simulink model "Simulation"  (R2015b)
settings: Solver=VariableStepAuto  StartTime=0.0  StopTime=10  RelTol=1e-3
undefined symbols (not defined in the file or in its folder): sigbuilder_block
settings Model: Creator=TOSHIBA  LastModifiedBy=TOSHIBA

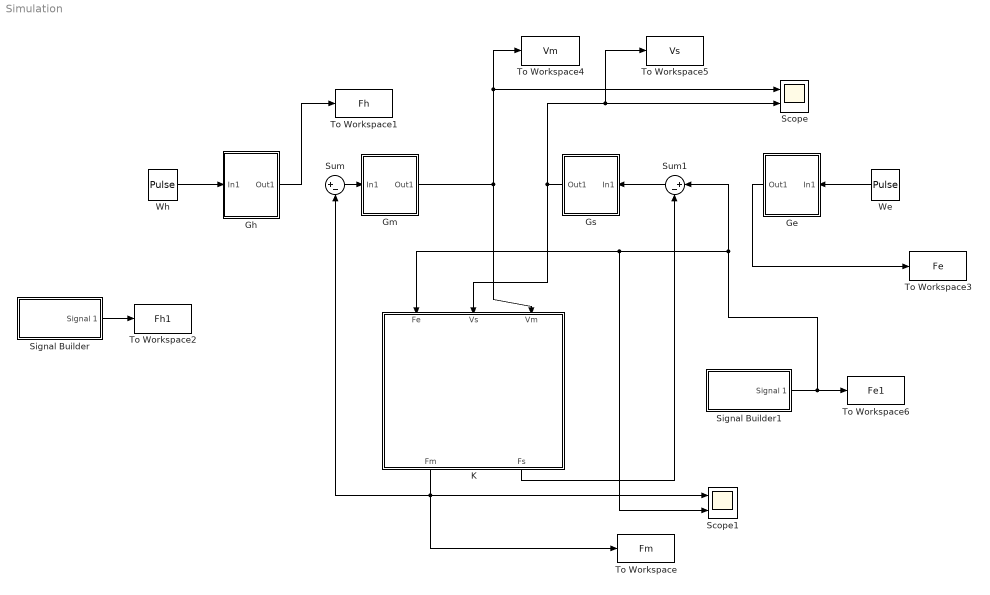
== system Simulation ==
  Ge : Subsystem
  Gh : Subsystem
  Gm : Subsystem
  Gs : Subsystem
  K : Subsystem
  Scope : Scope  NumInputPorts=2
  Scope1 : Scope  NumInputPorts=2
  Signal Builder : Subsystem  Tag=STV Subsys  LoadFcn=sigbuilder_block('load');  StartFcn=sigbuilder_block('start');  StopFcn=sigbuilder_block('stop');  ClipboardFcn=sigbuilder_block('clipboard');  mask(Sigbuilder block){}
      mask help: Simulink:masks:SigbuilderBlock_MD
      mask init:
      | if ~strcmp(get_param(bdroot(gcbh),'SimulationStatus'),'stopped') tuvar = sigbuilder_block('maskInit'); end
      settings: CopyFcn=sigbuilder_block('copy');  DeleteFcn=sigbuilder_block('delete');  ModelCloseFcn=sigbuilder_block('modelClose');  PreSaveFcn=sigbuilder_block('preSave');  PauseFcn=sigbuilder_block('pause');  ContinueFcn=sigbuilder_block('continue');  NameChangeFcn=sigbuilder_block('namechange');  OpenFcn=sigbuilder_block('open',[437.25 153.75 550.5 358.5 ]);  CloseFcn=sigbuilder_block('close');
      mask Display: plot(0, 0, 100, 100,[2, 2, 32, 32, 2], [68, 8, 8, 68, 68],[32, 2], [38, 38], [32, 19, 2],[53, 60, 44], [32, 17, 17, 2],[16, 16, 31, 31]);txt = getActiveGroup(gcbh);text(2, 100, txt,'verticalAlignment', 'top');
  Signal Builder1 : Subsystem  Tag=STV Subsys  LoadFcn=sigbuilder_block('load');  StartFcn=sigbuilder_block('start');  StopFcn=sigbuilder_block('stop');  ClipboardFcn=sigbuilder_block('clipboard');  mask(Sigbuilder block){}
      mask help: Simulink:masks:SigbuilderBlock_MD
      mask init:
      | if ~strcmp(get_param(bdroot(gcbh),'SimulationStatus'),'stopped') tuvar = sigbuilder_block('maskInit'); end
      settings: CopyFcn=sigbuilder_block('copy');  DeleteFcn=sigbuilder_block('delete');  ModelCloseFcn=sigbuilder_block('modelClose');  PreSaveFcn=sigbuilder_block('preSave');  PauseFcn=sigbuilder_block('pause');  ContinueFcn=sigbuilder_block('continue');  NameChangeFcn=sigbuilder_block('namechange');  OpenFcn=sigbuilder_block('open',[437.25 153.75 550.5 358.5 ]);  CloseFcn=sigbuilder_block('close');
      mask Display: plot(0, 0, 100, 100,[2, 2, 32, 32, 2], [68, 8, 8, 68, 68],[32, 2], [38, 38], [32, 19, 2],[53, 60, 44], [32, 17, 17, 2],[16, 16, 31, 31]);txt = getActiveGroup(gcbh);text(2, 100, txt,'verticalAlignment', 'top');
  Sum : Sum  Inputs=|+-
  Sum1 : Sum  Inputs=|+-
  To Workspace : ToWorkspace  VariableName=Fm  SaveFormat=Structure With Time  SampleTime=-1
  To Workspace1 : ToWorkspace  VariableName=Fh  SaveFormat=Structure With Time  SampleTime=-1
  To Workspace2 : ToWorkspace  VariableName=Fh1  SaveFormat=Structure With Time  SampleTime=-1
  To Workspace3 : ToWorkspace  VariableName=Fe  SaveFormat=Structure With Time  SampleTime=-1
  To Workspace4 : ToWorkspace  VariableName=Vm  SaveFormat=Structure With Time  SampleTime=-1
  To Workspace5 : ToWorkspace  VariableName=Vs  SaveFormat=Structure With Time  SampleTime=-1
  To Workspace6 : ToWorkspace  VariableName=Fe1  SaveFormat=Structure With Time  SampleTime=-1
  We : DiscretePulseGenerator  PulseType=Time based  Amplitude=5000  Period=20  PulseWidth=0.001
  Wh : DiscretePulseGenerator  PulseType=Time based  Amplitude=50000000  Period=20  PulseWidth=0.0000001
  wires:
  Gm/1(Out1) -> To Workspace4/1, Scope/1, K/3(Vm)
  Gs/1(Out1) -> K/2(Vs), To Workspace5/1, Scope/2
  K/2(Fs) -> Sum1/2
  Sum/1 -> Gm/1(In1)
  K/1(Fm) -> To Workspace/1, Scope1/1, Sum/2
  Sum1/1 -> Gs/1(In1)
  We/1 -> Ge/1(In1)
  Signal Builder/1(Signal 1) -> To Workspace2/1
  Wh/1 -> Gh/1(In1)
  Gh/1(Out1) -> To Workspace1/1
  Signal Builder1/1(Signal 1) -> Scope1/2, K/1(Fe), Sum1/1, To Workspace6/1
  Ge/1(Out1) -> To Workspace3/1

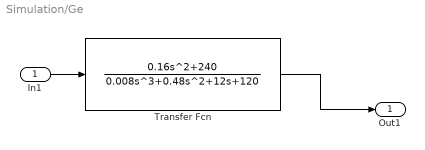
== system Simulation/Ge ==
  In1 : Inport
  Transfer Fcn : TransferFcn  Numerator=[0.16 0 240]  Denominator=[0.008 0.48 12 120]
  Out1 : Outport
  wires:
  In1/1 -> Transfer Fcn/1
  Transfer Fcn/1 -> Out1/1

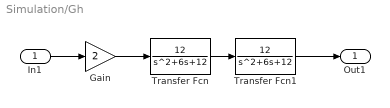
== system Simulation/Gh ==
  In1 : Inport
  Gain : Gain  Gain=2
  Transfer Fcn : TransferFcn  Numerator=[12]  Denominator=[1 6 12]
  Transfer Fcn1 : TransferFcn  Numerator=[12]  Denominator=[1 6 12]
  Out1 : Outport
  wires:
  Transfer Fcn/1 -> Transfer Fcn1/1
  In1/1 -> Gain/1
  Transfer Fcn1/1 -> Out1/1
  Gain/1 -> Transfer Fcn/1

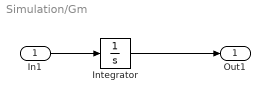
== system Simulation/Gm ==
  In1 : Inport
  Integrator : Integrator
  Out1 : Outport
  wires:
  Integrator/1 -> Out1/1
  In1/1 -> Integrator/1

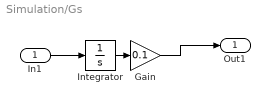
== system Simulation/Gs ==
  In1 : Inport
  Gain : Gain  Gain=0.1
  Integrator : Integrator
  Out1 : Outport
  wires:
  In1/1 -> Integrator/1
  Gain/1 -> Out1/1
  Integrator/1 -> Gain/1

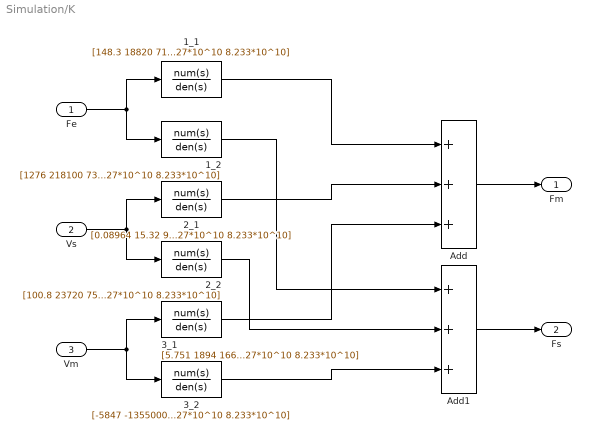
== system Simulation/K ==
  Fe : Inport
  Vs : Inport  Port=2
  Vm : Inport  Port=3
  1_1 : TransferFcn  Numerator=[148.3 18820 716100 3.695*10^7 5.545*10^8 4.28*10^9 1.985*10^10 5.593*10^10 7.853*10^10]  Denominator=[1 335.7 31020 1138000 4.555*10^7 6.604*10^8 4.954*10^9 2.22*10^10 6.027*10^10 8.233*10^10]
  1_2 : TransferFcn  Numerator=[1276 218100 7304000 3.914*10^8 4.397*10^9 2.309*10^10 6.563*10^10 1.053*10^11 8.622*10^10]  Denominator=[1 335.7 31020 1138000 4.555*10^7 6.604*10^8 4.954*10^9 2.22*10^10 6.027*10^10 8.233*10^10]
  2_1 : TransferFcn  Numerator=[0.08964 15.32 908 29960 394400 2858000 1.273*10^7 3.47*10^7 4.709*10^7]  Denominator=[1 335.7 31020 1138000 4.555*10^7 6.604*10^8 4.954*10^9 2.22*10^10 6.027*10^10 8.233*10^10]
  2_2 : TransferFcn  Numerator=[100.8 23720 750500 3.959*10^7 6.141*10^8 4.739*10^9 2.158*10^10 5.934*10^10 8.215*10^10]  Denominator=[1 335.7 31020 1138000 4.555*10^7 6.604*10^8 4.954*10^9 2.22*10^10 6.027*10^10 8.233*10^10]
  3_1 : TransferFcn  Numerator=[5.751 1894 166900 5602000 2.286*10^8 2.508*10^9 1.306*10^10 3.533*10^10 4.325*10^10]  Denominator=[1 335.7 31020 1138000 4.555*10^7 6.604*10^8 4.954*10^9 2.22*10^10 6.027*10^10 8.233*10^10]
  3_2 : TransferFcn  Numerator=[-5847 -1355000 -3.831*10^7 -2.155*10^9 -2.756*10^10 -1.678*10^11 -5.494*10^11 -8.528*10^11 -7.986*10^10]  Denominator=[1 335.7 31020 1138000 4.555*10^7 6.604*10^8 4.954*10^9 2.22*10^10 6.027*10^10 8.233*10^10]
  Add : Sum  Inputs=+++
  Add1 : Sum  Inputs=+++
  Fm : Outport
  Fs : Outport  Port=2
  wires:
  Vm/1 -> 3_2/1, 3_1/1
  Vs/1 -> 2_1/1, 2_2/1
  2_1/1 -> Add/2
  Fe/1 -> 1_2/1, 1_1/1
  1_2/1 -> Add1/1
  2_2/1 -> Add1/2
  3_2/1 -> Add1/3
  Add1/1 -> Fs/1
  Add/1 -> Fm/1
  1_1/1 -> Add/1
  3_1/1 -> Add/3

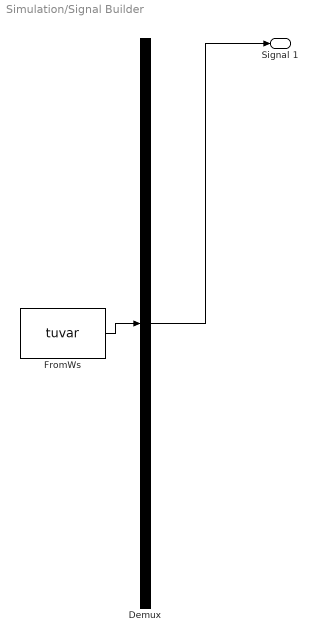
== system Simulation/Signal Builder ==
  Demux : Demux  Tag=STV Demux  Outputs=1
  FromWs : FromWorkspace  Tag=STV FromWs  VariableName=tuvar  SampleTime=0
      SigBuilderData=|
      | common.afterFinalStr = 'Extrapolate'
      | common.sampleTime = 0
      | dataSet.timeRange = [0 10]
      | dataSet.name = 'Group 1'
      | sbobj.Groups.Name = 'Group 1'
      | sbobj.Groups.Signals.Name = 'Signal 1'
      | sbobj.Groups.Signals.XData = [0 1 2 6 10]
      | sbobj.Groups.Signals.YData = [0 2 0 0 0]
  Signal 1 : Outport  Tag=STV Outport
  wires:
  Demux/1 -> Signal 1/1
  FromWs/1 -> Demux/1

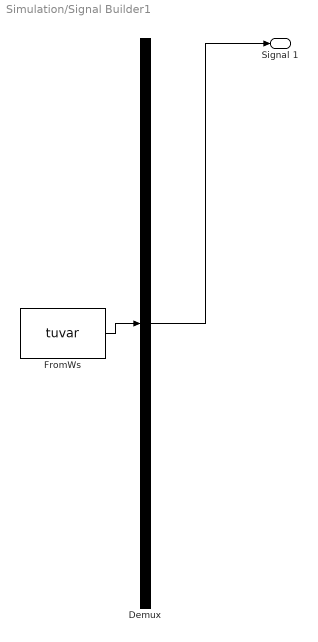
== system Simulation/Signal Builder1 ==
  Demux : Demux  Tag=STV Demux  Outputs=1
  FromWs : FromWorkspace  Tag=STV FromWs  VariableName=tuvar  SampleTime=0
      SigBuilderData=|
      | common.afterFinalStr = 'Extrapolate'
      | common.sampleTime = 0
      | dataSet.timeRange = [0 10]
      | dataSet.name = 'Group 1'
      | sbobj.Groups.Name = 'Group 1'
      | sbobj.Groups.Signals.Name = 'Signal 1'
      | sbobj.Groups.Signals.XData = [0 0.2 0.2 6 10]
      | sbobj.Groups.Signals.YData = [10 10 0 0 0]
  Signal 1 : Outport  Tag=STV Outport
  wires:
  FromWs/1 -> Demux/1
  Demux/1 -> Signal 1/1
